simulink model "CAT797_lateral_dynamics_differential_flatness_control"  (R2026a)
settings: Solver=ode4  StopTime=sim_t  FixedStep=0.0001
PreLoadFcn:
  | addpath("G:\Control_Research\Autonomy_Mining_Dump_Truck\src\plant_model\lib")
values from neighbouring files (symbols this model uses):
  Cf = 5047000.0    [CAT_797F.sldd]
  Cr = 5047000.0    [CAT_797F.sldd]
  Iz = 7190000.0    [CAT_797F.sldd]
  k0 = 3.0    [CAT_797F.sldd]
  k1 = 3.8    [CAT_797F.sldd]
  ki = 0.2    [CAT_797F.sldd]
  ky = 1.5    [CAT_797F.sldd]
  Lf = 2.5    [CAT_797F.sldd]
  Lr = 2.3    [CAT_797F.sldd]
libraries: simulink_extras x1, lat_dyn_haul_00 x1
settings Model: DataDictionary=CAT_797F.sldd  Creator=marti343  LastModifiedBy=USER
settings OptimizationCC: EnableMemcpy=off
settings HardwareCC: ProdBitPerChar=16.0  ProdBitPerInt=16.0  ProdLargestAtomicInteger=Integer  ProdWordSize=16.0  ProdHWDeviceType=Texas Instruments->C2000
settings RTWCC: GenerateReport=on  LaunchReport=on
settings CodeAppCC: MATLABSourceComments=on

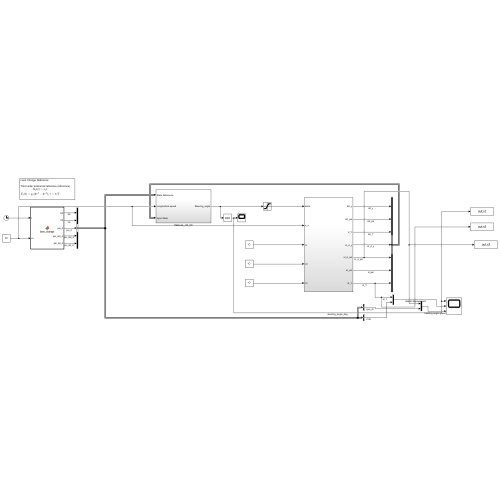
[thumbnail: Simulink's stored preview of the top-level diagram]
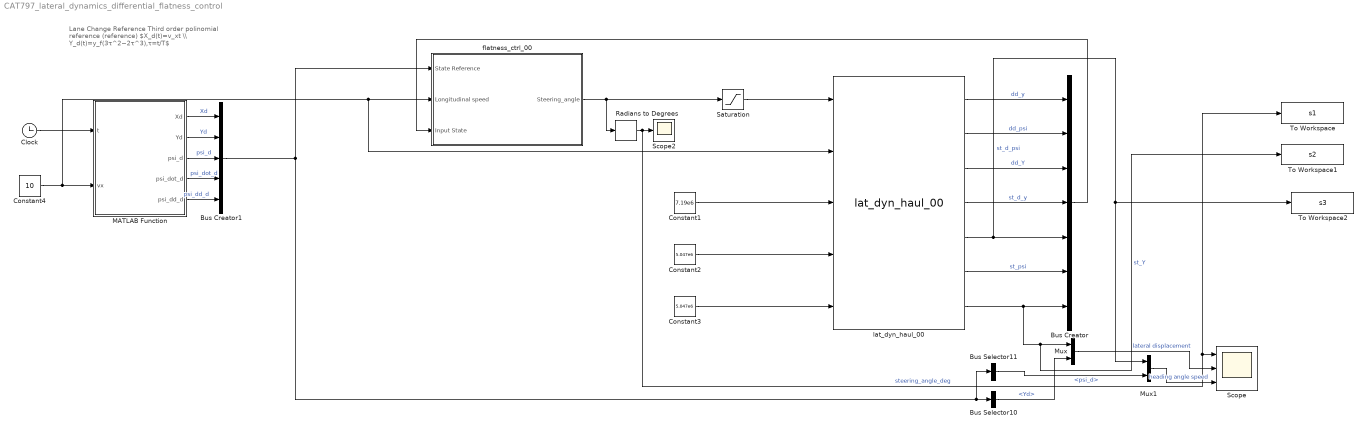
== system CAT797_lateral_dynamics_differential_flatness_control ==
  note: Lane Change Reference
      |
      | Third order polinomial reference (reference)
      | $X_d​(t)=v_x​t \\ Y_d(t)=y_f(3τ^2−2τ^3),τ=t/T$
  Bus Creator : BusCreator  Inputs=7
  Bus Creator1 : BusCreator  Inputs=5
  Bus Selector10 : BusSelector  OutputSignals=Yd
  Bus Selector11 : BusSelector  OutputSignals=psi_d
  Clock : Clock
  Constant1 : Constant  Value=7.19e6
  Constant2 : Constant  Value=5.047e6
  Constant3 : Constant  Value=5.047e6
  Constant4 : Constant  Value=10
  MATLAB Function : MATLAB Function  TreatAsAtomicUnit=on
  Mux : Mux  Inputs=2
  Mux1 : Mux  Inputs=2
  Radians to Degrees : simulink_extras/Transformations/Radians to Degrees
  Saturation : Saturate  UpperLimit=25  LowerLimit=-25
  Scope : Scope  NumInputPorts=3
      settings: ActiveDisplayString=3  ActiveDisplayYMinimum=-0.0065564806544863869  ActiveDisplayYMaximum=0.059008325890377494
  Scope2 : Scope
      settings: ActiveDisplayYMinimum=-1  ActiveDisplayYMaximum=1  DataLoggingVariableName=ScopeData2
  To Workspace : ToWorkspace  VariableName=s1  SaveFormat=Timeseries  SampleTime=-1
  To Workspace1 : ToWorkspace  VariableName=s2  SaveFormat=Timeseries  SampleTime=-1
  To Workspace2 : ToWorkspace  VariableName=s3  SaveFormat=Timeseries  SampleTime=-1
  flatness_ctrl_00 : Subsystem
  lat_dyn_haul_00 : lat_dyn_haul_00/lat_dyn_haul_00  SystemSampleTime=-1  VariantActivationTime=update diagram  EmptyChoice=off  PassThrough=off  PassThroughVariantControl=(default)  EmptyChoiceVariantControl=(default)  AllowFlexibleInterface=on  Latency=0  AutoFrameSizeCalculation=off
  wires:
  lat_dyn_haul_00/1 -> Bus Creator/1  "dd_y"
  lat_dyn_haul_00/3 -> Bus Creator/3  "dd_Y"
  lat_dyn_haul_00/4 -> Bus Creator/4  "st_d_y"
  Constant4/1 -> lat_dyn_haul_00/2, flatness_ctrl_00/2(Longitudinal speed), MATLAB Function/2(vx)
  Constant1/1 -> lat_dyn_haul_00/3
  Constant2/1 -> lat_dyn_haul_00/4
  Constant3/1 -> lat_dyn_haul_00/5
  Saturation/1 -> lat_dyn_haul_00/1
  lat_dyn_haul_00/2 -> Bus Creator/2  "dd_psi"
  lat_dyn_haul_00/6 -> Bus Creator/6  "st_psi"
  lat_dyn_haul_00/7 -> To Workspace1/1, Mux/1, Bus Creator/7  "st_Y"
  Clock/1 -> MATLAB Function/1(t)
  MATLAB Function/1(Xd) -> Bus Creator1/1  "Xd"
  MATLAB Function/2(Yd) -> Bus Creator1/2  "Yd"
  MATLAB Function/3(psi_d) -> Bus Creator1/3  "psi_d"
  MATLAB Function/4(psi_dot_d) -> Bus Creator1/4  "psi_dot_d"
  MATLAB Function/5(psi_dd_d) -> Bus Creator1/5  "psi_dd_d"
  Bus Creator1/1 -> flatness_ctrl_00/1(State Reference), Bus Selector11/1, Bus Selector10/1
  Bus Selector10/1 -> Mux/2  "<Yd>"
  Bus Selector11/1 -> Mux1/2  "<psi_d>"
  lat_dyn_haul_00/5 -> Mux1/1, To Workspace2/1, Bus Creator/5  "st_d_psi"
  Bus Creator/1 -> flatness_ctrl_00/3(Input State)
  flatness_ctrl_00/1(Steering_angle) -> Radians to Degrees/1, Saturation/1
  Radians to Degrees/1 -> To Workspace/1, Scope/1, Scope2/1  "steering_angle_deg"
  Mux/1 -> Scope/2  "lateral displacement"
  Mux1/1 -> Scope/3  "heading angle speed"

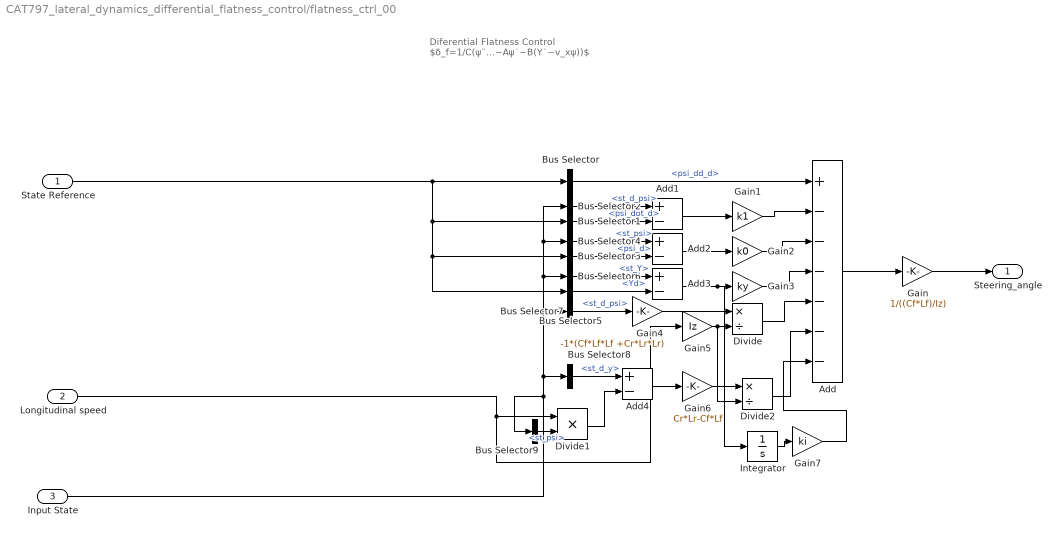
== system CAT797_lateral_dynamics_differential_flatness_control/flatness_ctrl_00 ==
  note: Diferential Flatness Control
      |
      | $δ_f​=1/C​(ψ¨_d​−k_1​(ψ˙​−ψ˙​_d​)−k_0​(ψ−ψ_d​)−k_y​e_y​−Aψ˙​−B(Y˙−v_x​ψ))$
  State Reference : Inport
  Longitudinal speed : Inport  Port=2
  Input State : Inport  Port=3
  Add : Sum  Inputs=+------
  Add{1..4} (4 alike) : Sum  Inputs=+-
  Bus Selector : BusSelector  OutputSignals=psi_dd_d
  Bus Selector1 : BusSelector  OutputSignals=psi_dot_d
  Bus Selector2 : BusSelector  OutputSignals=st_d_psi
  Bus Selector3 : BusSelector  OutputSignals=psi_d
  Bus Selector4 : BusSelector  OutputSignals=st_psi
  Bus Selector5 : BusSelector  OutputSignals=Yd
  Bus Selector6 : BusSelector  OutputSignals=st_Y
  Bus Selector7 : BusSelector  OutputSignals=st_d_psi
  Bus Selector8 : BusSelector  OutputSignals=st_d_y
  Bus Selector9 : BusSelector  OutputSignals=st_psi
  Divide : Product  Inputs=*/
  Divide1 : Product  Inputs=**
  Divide2 : Product  Inputs=*/
  Gain : Gain  Gain=1/((Cf*Lf)/Iz)
  Gain1 : Gain  Gain=k1
  Gain2 : Gain  Gain=k0
  Gain3 : Gain  Gain=ky
  Gain4 : Gain  Gain=-1*(Cf*Lf*Lf +Cr*Lr*Lr)
  Gain5 : Gain  Gain=Iz
  Gain6 : Gain  Gain=Cr*Lr-Cf*Lf
  Gain7 : Gain  Gain=ki
  Integrator : Integrator
  Steering_angle : Outport
  wires:
  Add/1 -> Gain/1
  Gain2/1 -> Add/3
  Add3/1 -> Integrator/1, Gain3/1
  Divide1/1 -> Add4/2
  Divide2/1 -> Add/6
  Input State/1 -> Bus Selector2/1, Bus Selector4/1, Bus Selector6/1, Bus Selector7/1, Bus Selector8/1, Bus Selector9/1
  State Reference/1 -> Bus Selector5/1, Bus Selector3/1, Bus Selector1/1, Bus Selector/1
  Gain5/1 -> Divide2/2, Divide/2
  Bus Selector7/1 -> Gain4/1  "<st_d_psi>"
  Bus Selector4/1 -> Add2/1  "<st_psi>"
  Bus Selector1/1 -> Add1/2  "<psi_dot_d>"
  Bus Selector5/1 -> Add3/2  "<Yd>"
  Bus Selector9/1 -> Divide1/2  "<st_psi>"
  Gain7/1 -> Add/7
  Gain1/1 -> Add/2
  Add2/1 -> Gain2/1
  Gain/1 -> Steering_angle/1
  Gain3/1 -> Add/4
  Bus Selector6/1 -> Add3/1  "<st_Y>"
  Add1/1 -> Gain1/1
  Bus Selector3/1 -> Add2/2  "<psi_d>"
  Longitudinal speed/1 -> Gain5/1, Divide1/1
  Integrator/1 -> Gain7/1
  Bus Selector/1 -> Add/1  "<psi_dd_d>"
  Bus Selector2/1 -> Add1/1  "<st_d_psi>"
  Add4/1 -> Gain6/1
  Bus Selector8/1 -> Add4/1  "<st_d_y>"
  Divide/1 -> Add/5
  Gain6/1 -> Divide2/1
  Gain4/1 -> Divide/1

== matlab function CAT797_lateral_dynamics_differential_flatness_control/MATLAB Function ==
  data: t input; Xd output; vx input; Yd output; psi_d output; psi_dot_d output; psi_dd_d output
function [Xd, Yd, psi_d, psi_dot_d, psi_dd_d] = lane_change(t, vx)

% PARAMETERS (tune these)
T  = 10;       % duration [s]
yf = 3.5;      % lateral shift [m]

% Normalize time
tau = t / T;

% Clamp tau between 0 and 1
if tau > 1
    tau = 1;
end
if tau < 0
    tau = 0;
end

% =========================
% POSITION
% =========================
Xd = vx * t;
Yd = yf * (3*tau^2 - 2*tau^3);

% =========================
% FIRST DERIVATIVE
% =========================
Xd_dot = vx;
Yd_dot = yf * (6*tau/T - 6*tau^2/T);

% =========================
% SECOND DERIVATIVE
% =========================
Xd_ddot = 0;
Yd_ddot = yf * (6/T^2 - 12*tau/T^2);

% =========================
% HEADING
% =========================
psi_d = atan2(Yd_dot, Xd_dot);

% =========================
% YAW RATE
% =========================
psi_dot_d = (Xd_dot * Yd_ddot - Yd_dot * Xd_ddot) / ...
            (Xd_dot^2 + Yd_dot^2);

% =========================
% YAW ACCELERATION (optional)
% =========================
% Numerical approximation (simple)
dt = 1e-3;

tau2 = (t+dt)/T;
if tau2 > 1
    tau2 = 1;
end

Yd_dot_2 = yf * (6*tau2/T - 6*tau2^2/T);
psi_d_2 = atan2(Yd_dot_2, vx);

psi_dd_d = (psi_d_2 - psi_d) / dt;

end
